simulink model "Innerloop_joystick_PIL_N1(1)"  (R2015a)
settings: Solver=ode45  StartTime=0.0  StopTime=100  FixedStep=0.01  RelTol=1e-3
undefined symbols (not defined in the file or in its folder): kdp, kdps, kdt, kdz, kpp, kpps, kpt, kpz
libraries: aerolibutil x2, vrlib x2
settings Model: Creator=abdelrazzak.merheb  LastModifiedBy=flying
settings DataIOCC: SignalLoggingSaveFormat=ModelDataLogs
settings OptimizationCC: ExpressionDepthLimit=2147483647
settings DebuggingCC: UnderspecifiedInitializationDetection=Classic  MergeDetectMultiDrivingBlocksExec=none  SolverPrmCheckMsg=warning  FcnCallInpInsideContextMsg=UseLocalSettings  StateNameClashWarn=warning
settings GRTTargetCC: CombineOutputUpdateFcns=off  GRTInterface=on

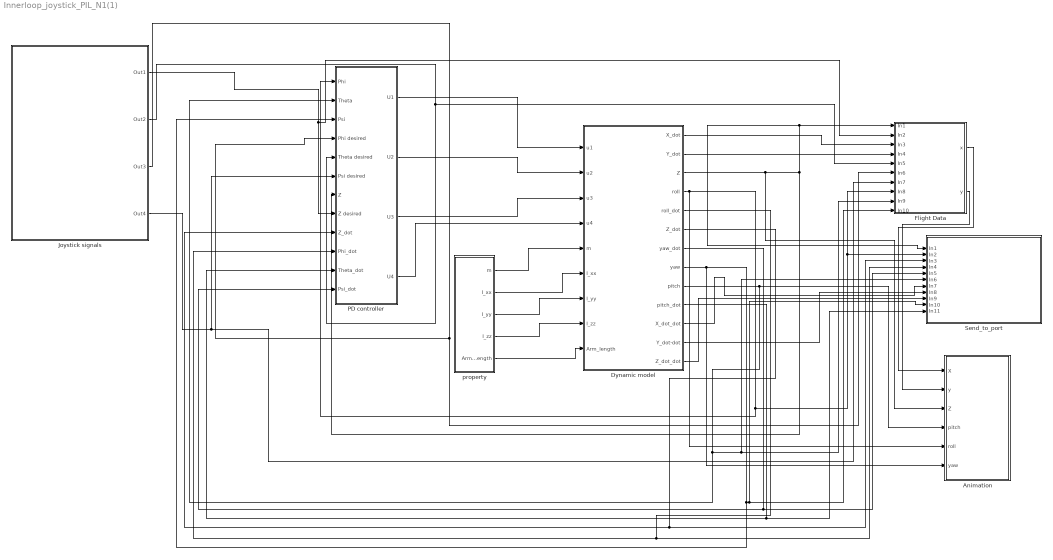
== system Innerloop_joystick_PIL_N1(1) ==
  "Animation " : Subsystem
  Dynamic model : Subsystem
  Flight Data : Subsystem
  Joystick signals : Subsystem
  PD controller : Subsystem
  Send_to_port : Subsystem
  "property " : Subsystem
  wires:
  Dynamic model/9(pitch) -> "Animation "/4(pitch), PD controller/2(Theta), Send_to_port/6(In6), Flight Data/9(In9)
  Dynamic model/3(Z) -> "Animation "/3(Z), PD controller/7(Z), Send_to_port/1(In1), Flight Data/1(In1)
  Dynamic model/4(roll) -> "Animation "/5(roll), PD controller/1(Phi), Send_to_port/2(In2), Flight Data/8(In8)
  Dynamic model/6(Z_dot) -> Send_to_port/3(In3), PD controller/9(Z_dot)
  Dynamic model/5(roll_dot) -> Send_to_port/4(In4), PD controller/10(Phi_dot)
  Dynamic model/10(pitch_dot) -> Send_to_port/11(In11), PD controller/11(Theta_dot)
  Dynamic model/7(yaw_dot) -> Send_to_port/5(In5), PD controller/12("Psi_dot ")
  Dynamic model/8(yaw) -> "Animation "/6(yaw), PD controller/3(Psi), Send_to_port/10(In10), Flight Data/10(In10)
  Dynamic model/11(X_dot_dot) -> Send_to_port/7(In7)
  Dynamic model/12(Y_dot-dot) -> Send_to_port/8(In8)
  Dynamic model/13(Z_dot_dot) -> Send_to_port/9(In9)
  Joystick signals/4(Out4) -> Flight Data/7(In7), PD controller/6(Psi desired)
  Joystick signals/3(Out3) -> Flight Data/6(In6), PD controller/4(Phi desired)
  Joystick signals/2(Out2) -> PD controller/5(Theta desired), Flight Data/5(In5)
  Joystick signals/1(Out1) -> Flight Data/2(In2), PD controller/8(Z desired)
  Dynamic model/1("X_dot ") -> Flight Data/3(In3)
  Dynamic model/2(Y_dot) -> Flight Data/4(In4)
  "property "/5("Arm_length ") -> Dynamic model/9(Arm_length)
  "property "/4(I_zz) -> Dynamic model/8(I_zz)
  "property "/3(I_yy) -> Dynamic model/7(I_yy)
  "property "/2(I_xx) -> Dynamic model/6(I_xx)
  "property "/1(m) -> Dynamic model/5(m)
  PD controller/2(U2) -> Dynamic model/2(u2)
  PD controller/3(U3) -> Dynamic model/3(u3)
  PD controller/1(U1) -> Dynamic model/1(u1)
  PD controller/4(U4) -> Dynamic model/4(u4)
  Flight Data/1(x) -> "Animation "/1(X)
  Flight Data/2(y) -> "Animation "/2(y)

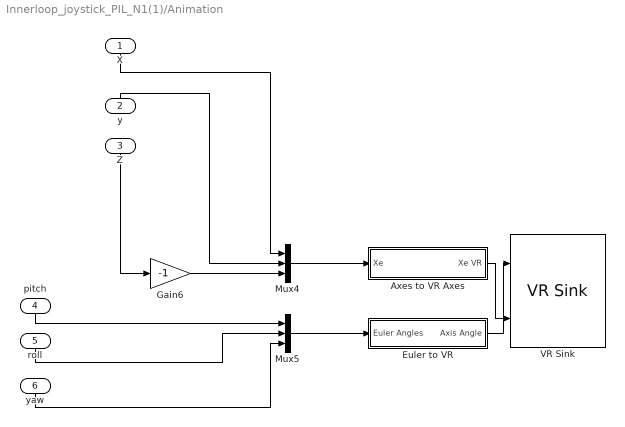
== system Innerloop_joystick_PIL_N1(1)/Animation  ==
  X : Inport
  y : Inport  Port=2
  Z : Inport  Port=3
  pitch : Inport  Port=4
  roll : Inport  Port=5
  yaw : Inport  Port=6
  Axes to VR Axes : Subsystem
  Euler to VR : Subsystem
  Gain6 : Gain  Gain=-1
  Mux4 : Mux  Inputs=3
  Mux5 : Mux  Inputs=3
  VR Sink : vrlib/VR Sink  InstantiateOnLoad=on  SampleTime=0.1  ViewEnable=on  RemoteChange=off  RemoteView=on  FieldsWritten=MyAirCraft.rotation.4.1.1.double#MyAirCraft.translation.3.1.1.double  WorldFileName=rollTst.wrl  AutoView=off  VideoDimensions=[]  AllowVariableSize=off
  wires:
  Mux5/1 -> Euler to VR/1(Euler Angles)
  Gain6/1 -> Mux4/3
  Axes to VR Axes/1(Xe VR) -> VR Sink/2
  Euler to VR/1(Axis Angle) -> VR Sink/1
  Mux4/1 -> Axes to VR Axes/1(Xe)
  yaw/1 -> Mux5/3
  roll/1 -> Mux5/2
  y/1 -> Mux4/2
  pitch/1 -> Mux5/1
  Z/1 -> Gain6/1
  X/1 -> Mux4/1

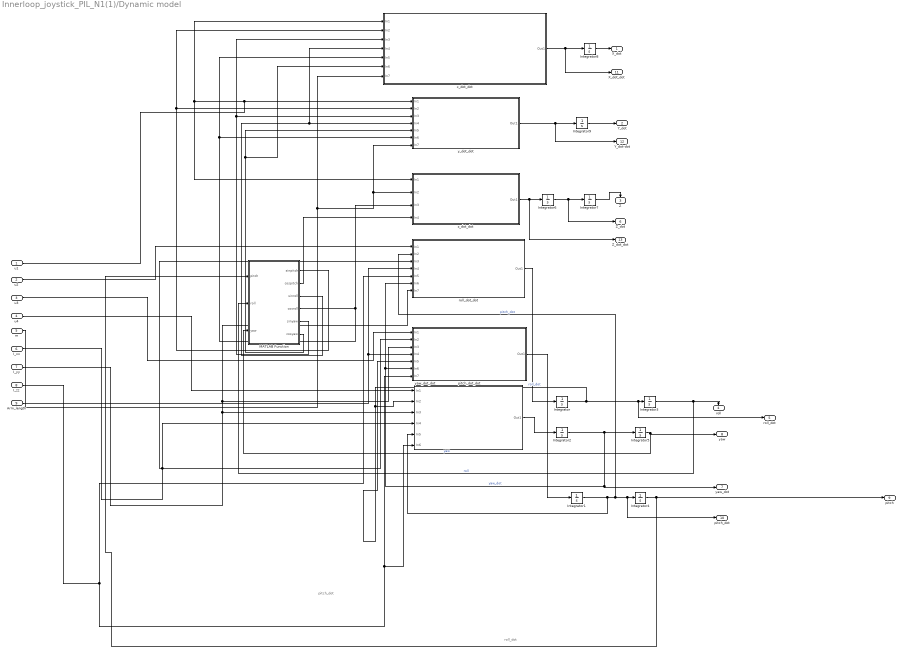
== system Innerloop_joystick_PIL_N1(1)/Dynamic model ==
  note: pitch_dot
  note: roll_dot
  u1 : Inport
  u2 : Inport  Port=2
  u3 : Inport  Port=3
  u4 : Inport  Port=4
  m : Inport  Port=5
  I_xx : Inport  Port=6
  I_yy : Inport  Port=7
  I_zz : Inport  Port=8
  Arm_length : Inport  Port=9
  Integrator{,1..9} (10 alike) : Integrator
  MATLAB Function : MATLAB Function  TreatAsAtomicUnit=on
  pitch_dot_dot : Subsystem
  roll_dot_dot : Subsystem
  x_dot_dot : Subsystem
  y_dot_dot : Subsystem
  yaw_dot_dot : Subsystem
  z_dot_dot : Subsystem
  "X_dot " : Outport
  Y_dot : Outport  Port=2
  Z : Outport  Port=3
  roll : Outport  Port=4
  roll_dot : Outport  Port=5
  Z_dot : Outport  Port=6
  yaw_dot : Outport  Port=7
  yaw : Outport  Port=8
  pitch : Outport  Port=9
  pitch_dot : Outport  Port=10
  X_dot_dot : Outport  Port=11
  Y_dot-dot : Outport  Port=12
  Z_dot_dot : Outport  Port=13
  wires:
  x_dot_dot/1(Out1) -> X_dot_dot/1, Integrator8/1
  Integrator6/1 -> Integrator7/1, Z_dot/1
  u4/1 -> yaw_dot_dot/1(In1)
  MATLAB Function/6(cosyaw) -> x_dot_dot/6(In6), y_dot_dot/5(In5)
  MATLAB Function/3(sinroll) -> x_dot_dot/4(In4), y_dot_dot/4(In4)
  MATLAB Function/4(cosroll) -> x_dot_dot/5(In5), y_dot_dot/6(In6), z_dot_dot/3(In3)
  MATLAB Function/1(sinpitch) -> x_dot_dot/2(In2), y_dot_dot/2(In2)
  m/1 -> x_dot_dot/7(In7), z_dot_dot/2(In2), y_dot_dot/7(In7)
  MATLAB Function/5(sinyaw) -> x_dot_dot/3(In3), y_dot_dot/3(In3)
  u1/1 -> y_dot_dot/1(In1), x_dot_dot/1(In1), z_dot_dot/1(In1)
  I_xx/1 -> yaw_dot_dot/4(In4), roll_dot_dot/3(In3), pitch_dot_dot/2(In2)
  I_yy/1 -> yaw_dot_dot/3(In3), roll_dot_dot/7(In7), pitch_dot_dot/3(In3)
  I_zz/1 -> roll_dot_dot/5(In5), yaw_dot_dot/6(In6), pitch_dot_dot/7(In7)
  Integrator3/1 -> roll/1, MATLAB Function/2(roll)  "roll"
  Integrator1/1 -> yaw_dot_dot/5(In5), roll_dot_dot/2(In2), pitch_dot/1, Integrator4/1  "pitch_dot"
  Integrator2/1 -> roll_dot_dot/6(In6), pitch_dot_dot/6(In6), yaw_dot/1, Integrator5/1  "yaw_dot"
  Integrator/1 -> pitch_dot_dot/5(In5), yaw_dot_dot/2(In2), roll_dot/1, Integrator3/1  "roll_dot"
  Integrator8/1 -> "X_dot "/1
  Integrator9/1 -> Y_dot/1
  Integrator5/1 -> MATLAB Function/3(yaw), yaw/1  "yaw"
  z_dot_dot/1(Out1) -> Z_dot_dot/1, Integrator6/1
  roll_dot_dot/1(Out1) -> Integrator/1
  pitch_dot_dot/1(Out1) -> Integrator1/1
  MATLAB Function/2(cospitch) -> z_dot_dot/4(In4)
  u2/1 -> roll_dot_dot/1(In1)
  Arm_length/1 -> roll_dot_dot/4(In4), pitch_dot_dot/4(In4)
  u3/1 -> pitch_dot_dot/1(In1)
  y_dot_dot/1(Out1) -> Y_dot-dot/1, Integrator9/1
  Integrator4/1 -> pitch/1, MATLAB Function/1(pitch)
  Integrator7/1 -> Z/1
  yaw_dot_dot/1(Out1) -> Integrator2/1

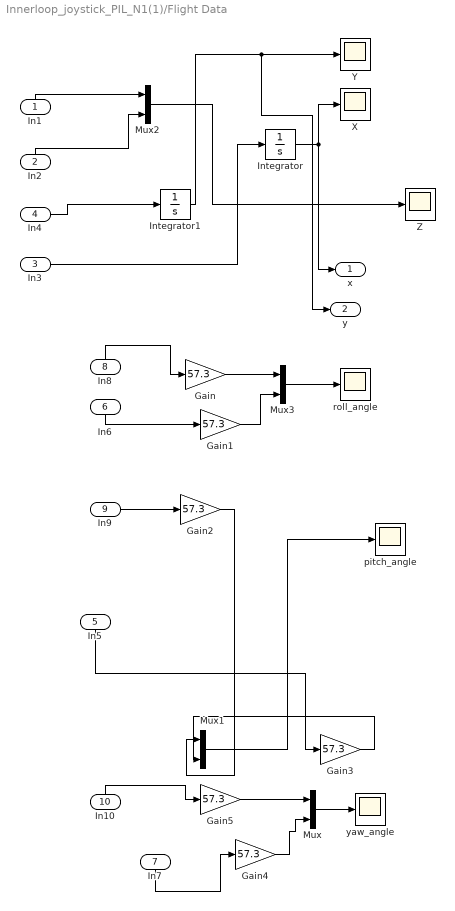
== system Innerloop_joystick_PIL_N1(1)/Flight Data ==
  In1 : Inport
  In2 : Inport  Port=2
  In3 : Inport  Port=3
  In4 : Inport  Port=4
  In5 : Inport  Port=5
  In6 : Inport  Port=6
  In7 : Inport  Port=7
  In8 : Inport  Port=8
  In9 : Inport  Port=9
  In10 : Inport  Port=10
  Gain{,1..5} (6 alike) : Gain  Gain=57.3
  Integrator : Integrator
  Integrator1 : Integrator
  Mux{,1..3} (4 alike) : Mux  Inputs=2
  X : Scope
      settings: YMin=-220  YMax=-160
  Y : Scope
      settings: YMin=-53000  YMax=-50750  SaveName=ScopeData2
  Z : Scope
      settings: YMin=95  YMax=105  SaveName=ScopeData3
  pitch_angle : Scope
  roll_angle : Scope
      settings: YMin=-7  YMax=12  SaveName=ScopeData4
  yaw_angle : Scope
      settings: YMin=2.5  YMax=8.5  SaveName=ScopeData5
  x : Outport
  y : Outport  Port=2
  wires:
  In2/1 -> Mux2/2
  In1/1 -> Mux2/1
  In10/1 -> Gain5/1
  In9/1 -> Gain2/1
  In6/1 -> Gain1/1
  In7/1 -> Gain4/1
  In5/1 -> Gain3/1
  In8/1 -> Gain/1
  In4/1 -> Integrator1/1
  In3/1 -> Integrator/1
  Gain/1 -> Mux3/1
  Gain4/1 -> Mux/2
  Mux2/1 -> Z/1
  Gain5/1 -> Mux/1
  Mux1/1 -> pitch_angle/1
  Gain2/1 -> Mux1/1
  Gain3/1 -> Mux1/2
  Mux/1 -> yaw_angle/1
  Mux3/1 -> roll_angle/1
  Integrator1/1 -> y/1, Y/1
  Gain1/1 -> Mux3/2
  Integrator/1 -> X/1, x/1

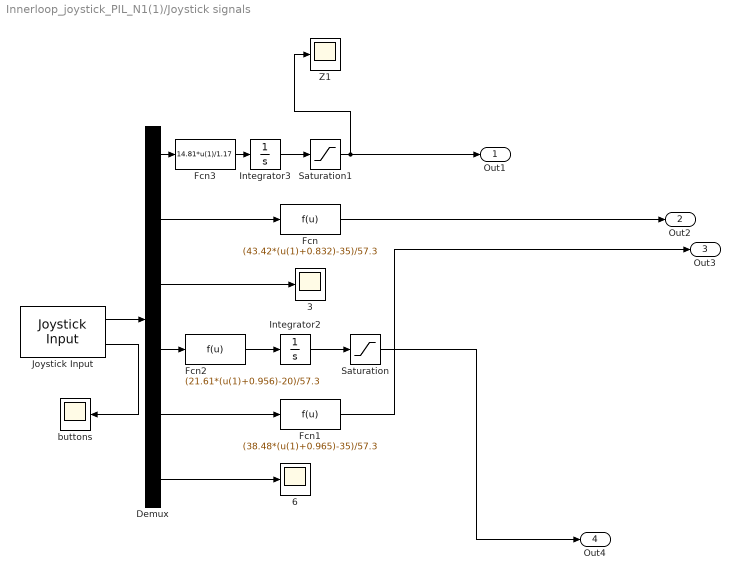
== system Innerloop_joystick_PIL_N1(1)/Joystick signals ==
  3 : Scope
      settings: SaveName=ScopeData9
  6 : Scope
      settings: SaveName=ScopeData10
  Demux : Demux  Outputs=6
  Fcn : Fcn  Expr=(43.42*(u(1)+0.832)-35)/57.3
  Fcn1 : Fcn  Expr=(38.48*(u(1)+0.965)-35)/57.3
  Fcn2 : Fcn  Expr=(21.61*(u(1)+0.956)-20)/57.3
  Fcn3 : Fcn  Expr=14.81*u(1)/1.17
  Integrator2 : Integrator
  Integrator3 : Integrator
  Joystick Input : vrlib/Joystick Input  joyid=1  adjustports=on  forcefeed=off
  Saturation : Saturate  UpperLimit=pi  LowerLimit=-pi
  Saturation1 : Saturate  UpperLimit=100  LowerLimit=0
  Z1 : Scope
      settings: YMin=-0.774  YMax=-0.765  SaveName=ScopeData7
  buttons : Scope
      settings: SaveName=ScopeData12
  Out1 : Outport
  Out2 : Outport  Port=2
  Out3 : Outport  Port=3
  Out4 : Outport  Port=4
  wires:
  Integrator2/1 -> Saturation/1
  Joystick Input/1 -> Demux/1
  Demux/1 -> Fcn3/1
  Demux/3 -> 3/1
  Demux/5 -> Fcn1/1
  Demux/2 -> Fcn/1
  Demux/6 -> 6/1
  Joystick Input/2 -> buttons/1
  Demux/4 -> Fcn2/1
  Fcn3/1 -> Integrator3/1
  Integrator3/1 -> Saturation1/1
  Fcn/1 -> Out2/1
  Fcn1/1 -> Out3/1
  Saturation/1 -> Out4/1
  Saturation1/1 -> Out1/1, Z1/1
  Fcn2/1 -> Integrator2/1

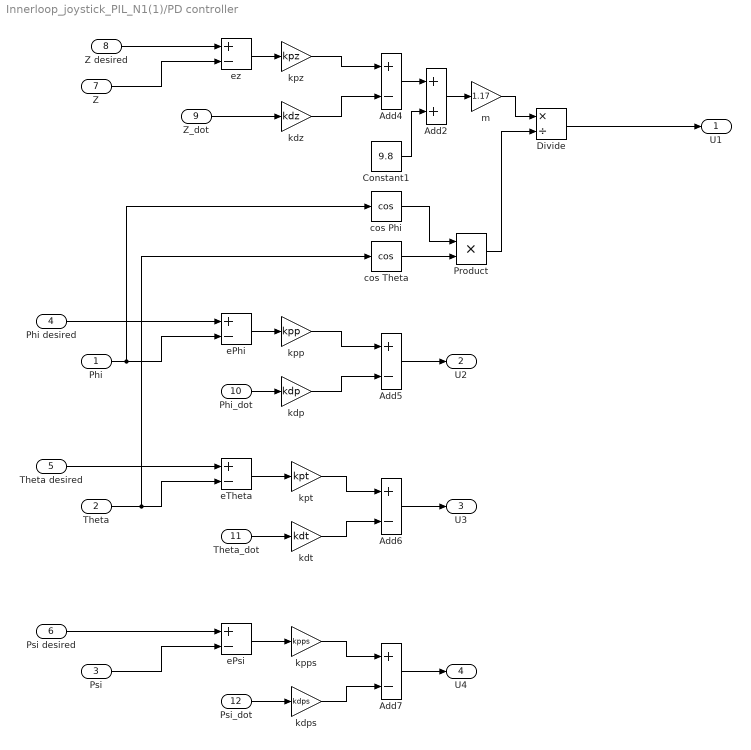
== system Innerloop_joystick_PIL_N1(1)/PD controller ==
  Phi : Inport
  Theta : Inport  Port=2
  Psi : Inport  Port=3
  Phi desired : Inport  Port=4
  Theta desired : Inport  Port=5
  Psi desired : Inport  Port=6
  Z : Inport  Port=7
  Z desired : Inport  Port=8
  Z_dot : Inport  Port=9
  Phi_dot : Inport  Port=10
  Theta_dot : Inport  Port=11
  "Psi_dot " : Inport  Port=12
  Add2 : Sum
  Add{4..7} (4 alike) : Sum  Inputs=+-
  Constant1 : Constant  Value=9.8
  Divide : Product  Inputs=*/
  Product : Product  RndMeth=Zero
  cos Phi : Trigonometry  Operator=cos
  cos Theta : Trigonometry  Operator=cos
  ePhi : Sum  Inputs=+-
  ePsi : Sum  Inputs=+-
  eTheta : Sum  Inputs=+-
  ez : Sum  Inputs=+-
  kdp : Gain  Gain=kdp
  kdps : Gain  Gain=kdps
  kdt : Gain  Gain=kdt
  kdz : Gain  Gain=kdz
  kpp : Gain  Gain=kpp
  kpps : Gain  Gain=kpps
  kpt : Gain  Gain=kpt
  kpz : Gain  Gain=kpz
  m : Gain  Gain=1.17
  U1 : Outport
  U2 : Outport  Port=2
  U3 : Outport  Port=3
  U4 : Outport  Port=4
  wires:
  Phi/1 -> ePhi/2, cos Phi/1
  Theta/1 -> eTheta/2, cos Theta/1
  Psi/1 -> ePsi/2
  Phi desired/1 -> ePhi/1
  Theta desired/1 -> eTheta/1
  Psi desired/1 -> ePsi/1
  ePhi/1 -> kpp/1
  Phi_dot/1 -> kdp/1
  eTheta/1 -> kpt/1
  Theta_dot/1 -> kdt/1
  ePsi/1 -> kpps/1
  "Psi_dot "/1 -> kdps/1
  Z desired/1 -> ez/1
  ez/1 -> kpz/1
  Z_dot/1 -> kdz/1
  kpz/1 -> Add4/1
  kdz/1 -> Add4/2
  kpp/1 -> Add5/1
  kdp/1 -> Add5/2
  Add5/1 -> U2/1
  kpt/1 -> Add6/1
  kdt/1 -> Add6/2
  Add6/1 -> U3/1
  kpps/1 -> Add7/1
  kdps/1 -> Add7/2
  Add7/1 -> U4/1
  cos Phi/1 -> Product/1
  cos Theta/1 -> Product/2
  m/1 -> Divide/1
  Product/1 -> Divide/2
  Divide/1 -> U1/1
  Add4/1 -> Add2/1
  Add2/1 -> m/1
  Constant1/1 -> Add2/2
  Z/1 -> ez/2

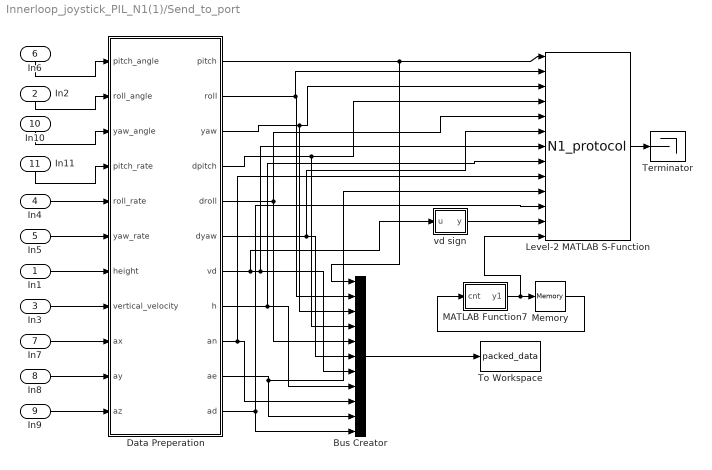
== system Innerloop_joystick_PIL_N1(1)/Send_to_port ==
  In1 : Inport
  In2 : Inport  Port=2
  In3 : Inport  Port=3
  In4 : Inport  Port=4
  In5 : Inport  Port=5
  In6 : Inport  Port=6
  In7 : Inport  Port=7
  In8 : Inport  Port=8
  In9 : Inport  Port=9
  In10 : Inport  Port=10
  In11 : Inport  Port=11
  Bus Creator : BusCreator  Inputs=11
  Data Preperation : MATLAB Function  TreatAsAtomicUnit=on
  Level-2 MATLAB S-Function : M-S-Function  FunctionName=N1_protocol
  MATLAB Function7 : MATLAB Function  TreatAsAtomicUnit=on
  Memory : Memory
  Terminator : Terminator
  To Workspace : ToWorkspace  VariableName=packed_data  SampleTime=-1
      settings: Save2DSignal=2-D array (concatenate along first dimension)
  vd sign : MATLAB Function  TreatAsAtomicUnit=on
  wires:
  Data Preperation/5(droll) -> Bus Creator/5, Level-2 MATLAB S-Function/5
  Data Preperation/10(ae) -> Level-2 MATLAB S-Function/10, Bus Creator/10
  In7/1 -> Data Preperation/9(ax)
  Data Preperation/6(dyaw) -> Level-2 MATLAB S-Function/6, Bus Creator/6
  Data Preperation/7(vd) -> vd sign/1(u), Level-2 MATLAB S-Function/7, Bus Creator/7
  Data Preperation/8(h) -> Level-2 MATLAB S-Function/8, Bus Creator/8
  Bus Creator/1 -> To Workspace/1
  Data Preperation/3(yaw) -> Level-2 MATLAB S-Function/3, Bus Creator/3
  Data Preperation/9(an) -> Level-2 MATLAB S-Function/9, Bus Creator/9
  Data Preperation/4(dpitch) -> Level-2 MATLAB S-Function/4, Bus Creator/4
  vd sign/1(y) -> Level-2 MATLAB S-Function/12
  MATLAB Function7/1(y1) -> Level-2 MATLAB S-Function/13, Memory/1
  Data Preperation/2(roll) -> Level-2 MATLAB S-Function/2, Bus Creator/2
  Level-2 MATLAB S-Function/1 -> Terminator/1
  In8/1 -> Data Preperation/10(ay)
  Data Preperation/11(ad) -> Bus Creator/11, Level-2 MATLAB S-Function/11
  Data Preperation/1(pitch) -> Bus Creator/1, Level-2 MATLAB S-Function/1
  In9/1 -> Data Preperation/11(az)
  Memory/1 -> MATLAB Function7/1(cnt)
  In5/1 -> Data Preperation/6(yaw_rate)
  In1/1 -> Data Preperation/7(height)
  In10/1 -> Data Preperation/3(yaw_angle)
  In6/1 -> Data Preperation/1(pitch_angle)
  In4/1 -> Data Preperation/5(roll_rate)
  In11/1 -> Data Preperation/4(pitch_rate)
  In3/1 -> Data Preperation/8(vertical_velocity)
  In2/1 -> Data Preperation/2(roll_angle)

== system Innerloop_joystick_PIL_N1(1)/property  ==
  Arm_length_ : Constant  Value=0.228
  ineretia_yy : Constant  Value=2.5955e-4
  inertia_xx : Constant  Value=2.754e-4
  inertia_zz : Constant  Value=5.7824e-5
  mass : Constant  Value=1.17
  m : Outport
  I_xx : Outport  Port=2
  I_yy : Outport  Port=3
  I_zz : Outport  Port=4
  "Arm_length " : Outport  Port=5
  wires:
  inertia_zz/1 -> I_zz/1
  Arm_length_/1 -> "Arm_length "/1
  ineretia_yy/1 -> I_yy/1
  mass/1 -> m/1
  inertia_xx/1 -> I_xx/1

== system Innerloop_joystick_PIL_N1(1)/Animation /Axes to VR Axes ==
  Xe : Inport
  Demux : Demux  Outputs=3
  Mux : Mux  Inputs=3
  rad-->deg : Gain  Gain=-1  SaturateOnIntegerOverflow=on  OutDataTypeStr=Inherit: Same as input  ParamDataTypeStr=Inherit: Same as input
  rad-->deg1 : Gain  Gain=-1  SaturateOnIntegerOverflow=on  OutDataTypeStr=Inherit: Same as input  ParamDataTypeStr=Inherit: Same as input
  Xe VR : Outport
  wires:
  Xe/1 -> Demux/1
  Demux/1 -> Mux/1
  Demux/2 -> rad-->deg/1
  Demux/3 -> rad-->deg1/1
  Mux/1 -> Xe VR/1
  rad-->deg1/1 -> Mux/2
  rad-->deg/1 -> Mux/3

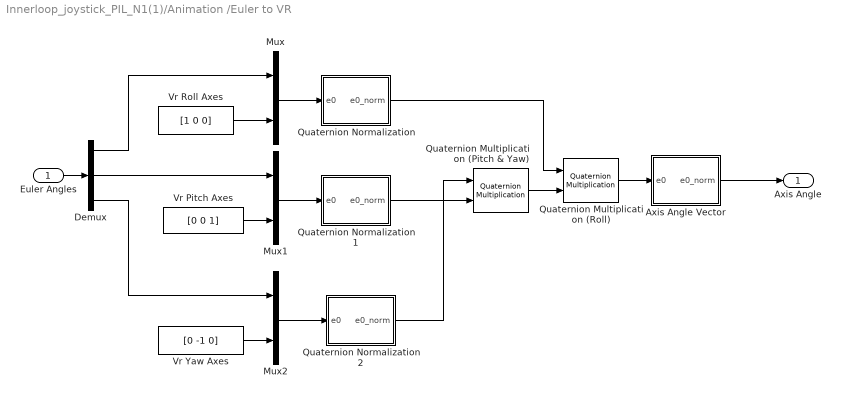
== system Innerloop_joystick_PIL_N1(1)/Animation /Euler to VR ==
  Euler Angles : Inport
  Axis Angle Vector : Subsystem
  Demux : Demux  Outputs=3
  Mux : Mux  Inputs=2
  Mux1 : Mux  Inputs=2
  Mux2 : Mux  Inputs=2
  Quaternion Multiplication (Pitch & Yaw) : aerolibutil/Quaternion Multiplication
  Quaternion Multiplication (Roll) : aerolibutil/Quaternion Multiplication
  Quaternion Normalization : Subsystem
  Quaternion Normalization1 : Subsystem
  Quaternion Normalization2 : Subsystem
  Vr Pitch Axes : Constant  Value=[0 0 1]
  Vr Roll Axes : Constant  Value=[1 0 0]
  Vr Yaw Axes : Constant  Value=[0 -1 0]
  Axis Angle : Outport
  wires:
  Quaternion Multiplication (Roll)/1 -> Axis Angle Vector/1(e0)
  Quaternion Multiplication (Pitch & Yaw)/1 -> Quaternion Multiplication (Roll)/2
  Axis Angle Vector/1(e0_norm) -> Axis Angle/1
  Quaternion Normalization/1(e0_norm) -> Quaternion Multiplication (Roll)/1
  Quaternion Normalization2/1(e0_norm) -> Quaternion Multiplication (Pitch & Yaw)/1
  Quaternion Normalization1/1(e0_norm) -> Quaternion Multiplication (Pitch & Yaw)/2
  Mux2/1 -> Quaternion Normalization2/1(e0)
  Mux1/1 -> Quaternion Normalization1/1(e0)
  Mux/1 -> Quaternion Normalization/1(e0)
  Demux/3 -> Mux2/1
  Vr Yaw Axes/1 -> Mux2/2
  Demux/2 -> Mux1/1
  Vr Pitch Axes/1 -> Mux1/2
  Demux/1 -> Mux/1
  Vr Roll Axes/1 -> Mux/2
  Euler Angles/1 -> Demux/1

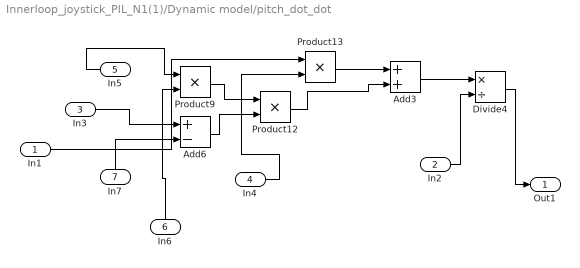
== system Innerloop_joystick_PIL_N1(1)/Dynamic model/pitch_dot_dot ==
  In1 : Inport
  In2 : Inport  Port=2
  In3 : Inport  Port=3
  In4 : Inport  Port=4
  In5 : Inport  Port=5
  In6 : Inport  Port=6
  In7 : Inport  Port=7
  Add3 : Sum
  Add6 : Sum  Inputs=+-
  Divide4 : Product  Inputs=*/
  Product12 : Product
  Product13 : Product
  Product9 : Product
  Out1 : Outport
  wires:
  Product12/1 -> Add3/2
  Product13/1 -> Add3/1
  In1/1 -> Product13/1
  Add6/1 -> Product12/2
  Add3/1 -> Divide4/1
  Product9/1 -> Product12/1
  In4/1 -> Product13/2
  In6/1 -> Product9/2
  In7/1 -> Add6/2
  In3/1 -> Add6/1
  In2/1 -> Divide4/2
  In5/1 -> Product9/1
  Divide4/1 -> Out1/1

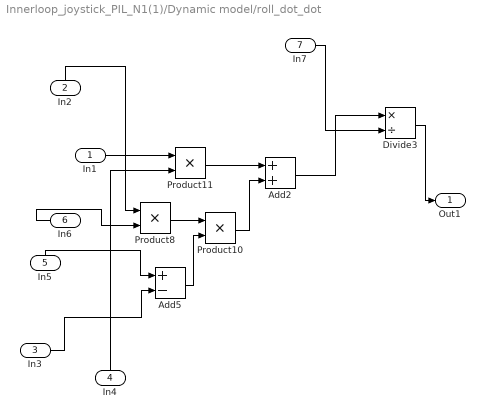
== system Innerloop_joystick_PIL_N1(1)/Dynamic model/roll_dot_dot ==
  In1 : Inport
  In2 : Inport  Port=2
  In3 : Inport  Port=3
  In4 : Inport  Port=4
  In5 : Inport  Port=5
  In6 : Inport  Port=6
  In7 : Inport  Port=7
  Add2 : Sum
  Add5 : Sum  Inputs=+-
  Divide3 : Product  Inputs=*/
  Product10 : Product
  Product11 : Product
  Product8 : Product
  Out1 : Outport
  wires:
  Product11/1 -> Add2/1
  Add5/1 -> Product10/2
  In1/1 -> Product11/1
  Add2/1 -> Divide3/1
  Product8/1 -> Product10/1
  Product10/1 -> Add2/2
  Divide3/1 -> Out1/1
  In5/1 -> Add5/1
  In3/1 -> Add5/2
  In2/1 -> Product8/1
  In7/1 -> Divide3/2
  In4/1 -> Product11/2
  In6/1 -> Product8/2

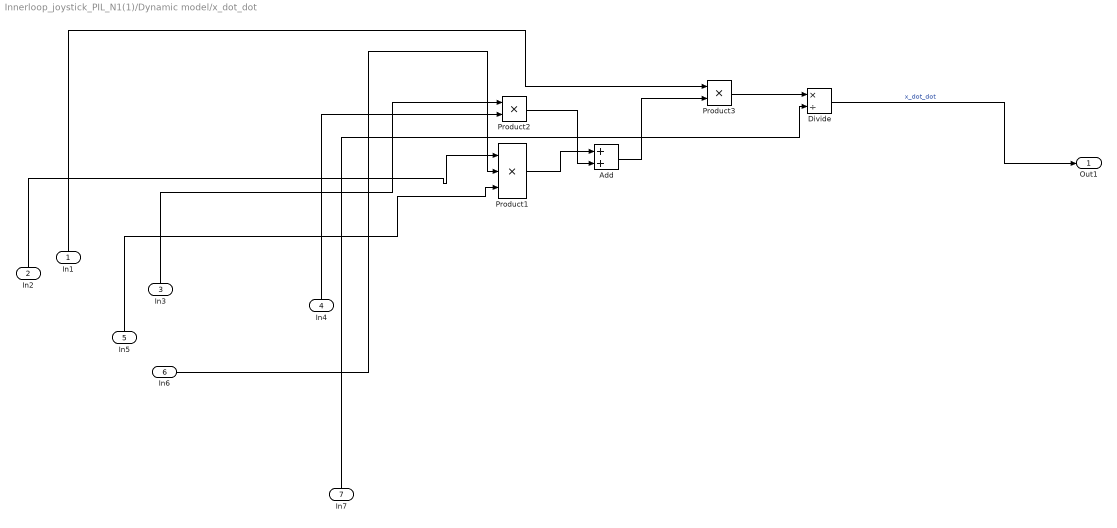
== system Innerloop_joystick_PIL_N1(1)/Dynamic model/x_dot_dot ==
  In1 : Inport
  In2 : Inport  Port=2
  In3 : Inport  Port=3
  In4 : Inport  Port=4
  In5 : Inport  Port=5
  In6 : Inport  Port=6
  In7 : Inport  Port=7
  Add : Sum
  Divide : Product  Inputs=*/
  Product1 : Product  Inputs=3
  Product2 : Product
  Product3 : Product
  Out1 : Outport
  wires:
  In1/1 -> Product3/1
  In6/1 -> Product1/2
  In7/1 -> Divide/2
  In4/1 -> Product2/2
  In3/1 -> Product2/1
  In5/1 -> Product1/3
  In2/1 -> Product1/1
  Divide/1 -> Out1/1  "x_dot_dot"
  Product2/1 -> Add/2
  Product1/1 -> Add/1
  Product3/1 -> Divide/1
  Add/1 -> Product3/2

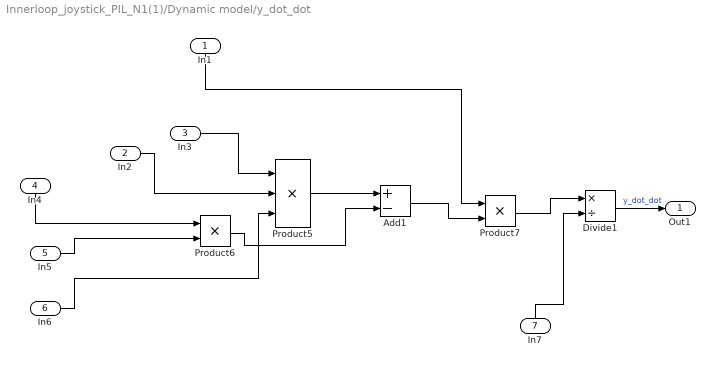
== system Innerloop_joystick_PIL_N1(1)/Dynamic model/y_dot_dot ==
  In1 : Inport
  In2 : Inport  Port=2
  In3 : Inport  Port=3
  In4 : Inport  Port=4
  In5 : Inport  Port=5
  In6 : Inport  Port=6
  In7 : Inport  Port=7
  Add1 : Sum  Inputs=+-
  Divide1 : Product  Inputs=*/
  Product5 : Product  Inputs=3
  Product6 : Product
  Product7 : Product
  Out1 : Outport
  wires:
  In1/1 -> Product7/1
  In2/1 -> Product5/2
  In5/1 -> Product6/2
  In7/1 -> Divide1/2
  In6/1 -> Product5/3
  In3/1 -> Product5/1
  In4/1 -> Product6/1
  Product5/1 -> Add1/1
  Add1/1 -> Product7/2
  Product6/1 -> Add1/2
  Divide1/1 -> Out1/1  "y_dot_dot"
  Product7/1 -> Divide1/1

== system Innerloop_joystick_PIL_N1(1)/Dynamic model/yaw_dot_dot ==
  In1 : Inport
  In2 : Inport  Port=2
  In3 : Inport  Port=3
  In4 : Inport  Port=4
  In5 : Inport  Port=5
  In6 : Inport  Port=6
  Add7 : Sum
  Add8 : Sum  Inputs=+-
  Divide5 : Product  Inputs=*/
  Product14 : Product
  Product15 : Product
  Out1 : Outport
  wires:
  In4/1 -> Add8/1
  In6/1 -> Divide5/2
  In2/1 -> Product15/2
  In3/1 -> Add8/2
  In5/1 -> Product15/1
  Product14/1 -> Add7/2
  Add8/1 -> Product14/2
  Product15/1 -> Product14/1
  In1/1 -> Add7/1
  Add7/1 -> Divide5/1
  Divide5/1 -> Out1/1

== system Innerloop_joystick_PIL_N1(1)/Dynamic model/z_dot_dot ==
  In1 : Inport
  In2 : Inport  Port=2
  In3 : Inport  Port=3
  In4 : Inport  Port=4
  Add4 : Sum  Inputs=-+
  Divide2 : Product  Inputs=*/
  Product : Product
  Product4 : Product
  u5 : Constant  Value=9.8
  Out1 : Outport
  wires:
  In3/1 -> Product4/2
  In2/1 -> Divide2/2
  In1/1 -> Product/2
  Divide2/1 -> Add4/2
  Product4/1 -> Product/1
  In4/1 -> Product4/1
  u5/1 -> Add4/1
  Product/1 -> Divide2/1
  Add4/1 -> Out1/1  "z_dot_dot"

== system Innerloop_joystick_PIL_N1(1)/Animation /Euler to VR/Axis Angle Vector ==
  e0 : Inport
  2 : Gain  Gain=2  SaturateOnIntegerOverflow=on  OutDataTypeStr=Inherit: Same as input  ParamDataTypeStr=Inherit: Same as input
  Concatenate : Concatenate
  Demux : Demux  Outputs=[1 3 ]
  Product : Product  Inputs=*/  SaturateOnIntegerOverflow=on  InputSameDT=on  OutDataTypeStr=Inherit: Same as first input
  Trigonometric Function : Trigonometry
  Trigonometric Function2 : Trigonometry  Operator=acos
  e0_norm : Outport
  wires:
  Demux/1 -> Trigonometric Function2/1
  Demux/2 -> Product/1
  Concatenate/1 -> e0_norm/1
  Product/1 -> Concatenate/1
  2/1 -> Concatenate/2
  Trigonometric Function/1 -> Product/2
  Trigonometric Function2/1 -> Trigonometric Function/1, 2/1
  e0/1 -> Demux/1

== system Innerloop_joystick_PIL_N1(1)/Animation /Euler to VR/Quaternion Normalization ==
  e0 : Inport
  1/2 : Gain  Gain=1/2  SaturateOnIntegerOverflow=on  OutDataTypeStr=Inherit: Same as input  ParamDataTypeStr=Inherit: Same as input
  Concatenate : Concatenate
  Demux : Demux  Outputs=[1 3]
  Product : Product  SaturateOnIntegerOverflow=on  InputSameDT=on  OutDataTypeStr=Inherit: Same as first input
  Trigonometric Function : Trigonometry
  Trigonometric Function1 : Trigonometry  Operator=cos
  e0_norm : Outport
  wires:
  Trigonometric Function1/1 -> Concatenate/1
  Demux/2 -> Product/2
  Demux/1 -> 1/2/1
  Concatenate/1 -> e0_norm/1
  Product/1 -> Concatenate/2
  Trigonometric Function/1 -> Product/1
  1/2/1 -> Trigonometric Function1/1, Trigonometric Function/1
  e0/1 -> Demux/1

== system Innerloop_joystick_PIL_N1(1)/Animation /Euler to VR/Quaternion Normalization1 ==
  e0 : Inport
  1/2 : Gain  Gain=1/2  SaturateOnIntegerOverflow=on  OutDataTypeStr=Inherit: Same as input  ParamDataTypeStr=Inherit: Same as input
  Concatenate : Concatenate
  Demux : Demux  Outputs=[1 3]
  Product : Product  SaturateOnIntegerOverflow=on  InputSameDT=on  OutDataTypeStr=Inherit: Same as first input
  Trigonometric Function : Trigonometry
  Trigonometric Function1 : Trigonometry  Operator=cos
  e0_norm : Outport
  wires:
  e0/1 -> Demux/1
  1/2/1 -> Trigonometric Function/1, Trigonometric Function1/1
  Trigonometric Function/1 -> Product/1
  Product/1 -> Concatenate/2
  Concatenate/1 -> e0_norm/1
  Demux/1 -> 1/2/1
  Demux/2 -> Product/2
  Trigonometric Function1/1 -> Concatenate/1

== system Innerloop_joystick_PIL_N1(1)/Animation /Euler to VR/Quaternion Normalization2 ==
  e0 : Inport
  1/2 : Gain  Gain=1/2  SaturateOnIntegerOverflow=on  OutDataTypeStr=Inherit: Same as input  ParamDataTypeStr=Inherit: Same as input
  Concatenate : Concatenate
  Demux : Demux  Outputs=[1 3]
  Product : Product  SaturateOnIntegerOverflow=on  InputSameDT=on  OutDataTypeStr=Inherit: Same as first input
  Trigonometric Function : Trigonometry
  Trigonometric Function1 : Trigonometry  Operator=cos
  e0_norm : Outport
  wires:
  Trigonometric Function1/1 -> Concatenate/1
  Demux/2 -> Product/2
  Demux/1 -> 1/2/1
  Concatenate/1 -> e0_norm/1
  Product/1 -> Concatenate/2
  Trigonometric Function/1 -> Product/1
  1/2/1 -> Trigonometric Function1/1, Trigonometric Function/1
  e0/1 -> Demux/1

== matlab function Innerloop_joystick_PIL_N1(1)/Send_to_port/vd sign ==
  data: u input; y output
function y = fcn(u)
if u>0;
y=bin2dec('00000000');
elseif u==0
y=bin2dec('00000000');
else u<0;
y=bin2dec('00000100');
end

== matlab function Innerloop_joystick_PIL_N1(1)/Send_to_port/Data Preperation ==
  data: pitch output; roll output; yaw output; pitch_angle input; roll_angle input; yaw_angle input; pitch_rate input; roll_rate input; yaw_rate input; dpitch output; droll output; dyaw output; vd output; h output; height input; an output; ae output; ad output; vertical_velocity input; ax input; ay input; az input
function [pitch,roll,yaw,dpitch,droll,dyaw,vd,h,an,ae,ad] = fcn(pitch_angle,roll_angle,yaw_angle,pitch_rate,roll_rate,yaw_rate,height,vertical_velocity,ax,ay,az)

pitch=round(pitch_angle*573);
roll=round(roll_angle*573);
yaw=round(yaw_angle*573);


dpitch=round(pitch_rate*573);
droll=round(roll_rate*573);
dyaw=round(yaw_rate*573);


h=round(height*1000);
vd=round(vertical_velocity*100);


Rotation_metrix=[
                  cos(pitch_angle)*cos(yaw_angle)-cos(roll_angle)*sin(pitch_angle)*sin(yaw_angle),-cos(roll_angle)*cos(yaw_angle)*sin(pitch_angle)-cos(pitch_angle)*sin(yaw_angle),sin(pitch_angle)*sin(roll_angle);
                  cos(yaw_angle)*sin(pitch_angle)+cos(pitch_angle)*cos(roll_angle)*sin(yaw_angle),cos(pitch_angle)*cos(roll_angle)-sin(pitch_angle)*sin(yaw_angle),-cos(pitch_angle)*sin(roll_angle);
                  sin(roll_angle)*sin(yaw_angle),cos(yaw_angle)*sin(roll_angle),cos(roll_angle)
];

B=[ax,ay,az]';
A=Rotation_metrix*B;
an=A(1,1);
ae=A(2,1);
ad=A(3,1);

an=round(an*100);
ae=round(ae*100);
ad=round(ad*100);

== matlab function Innerloop_joystick_PIL_N1(1)/Dynamic model/MATLAB Function ==
  data: pitch input; sinpitch output; roll input; yaw input; cospitch output; sinroll output; cosroll output; sinyaw output; cosyaw output
function [sinpitch,cospitch,sinroll,cosroll,sinyaw,cosyaw]= fcn(pitch,roll,yaw)
sinpitch=sin(pitch);
cospitch=cos(pitch);
sinroll=sin(roll);
cosroll=cos(roll);
sinyaw=sin(yaw);
cosyaw=cos(yaw);

== matlab function Innerloop_joystick_PIL_N1(1)/Send_to_port/MATLAB Function7 ==
  data: y1 output; cnt input
function y1= fcn(cnt)



y1=cnt+1;
if y1>255
y1=1;
end
